simulink model "GPSModel"  (R2017a)
settings: Solver=VariableStepAuto  StartTime=0.0  StopTime=10.0  RelTol=1e-3
undefined symbols (not defined in the file or in its folder): dpsV1, dpsV1seed, dpsV2, dpsV2seed, dpsV3, dpsV3seed, dpsV4, dpsV4seed, dpsV5, dpsV5seed, dpsV6, dpsV6seed, GPS_CLK, GpsClockBias, GpsClockDrift, TDI0, VI0, XI0
libraries: simulink x6
settings Model: Creator=AHKh  LastModifiedBy=AHKh

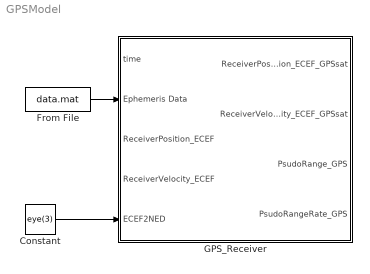
== system GPSModel ==
  Constant : Constant  Value=eye(3)
  From File : FromFile  FileName=data.mat  SampleTime=0
  GPS_Receiver : Subsystem
  wires:
  Constant/1 -> GPS_Receiver/5(ECEF2NED)
  From File/1 -> GPS_Receiver/2(Ephemeris Data)

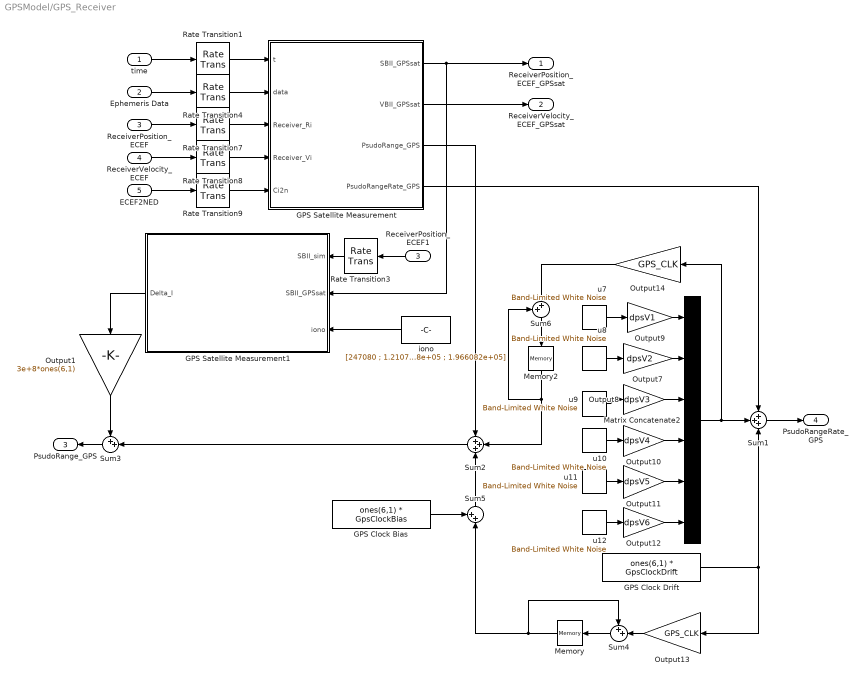
== system GPSModel/GPS_Receiver ==
  time : Inport  PortDimensions=[1,1]
  Ephemeris Data : Inport  Port=2
  ReceiverPosition_ECEF : Inport  Port=3  PortDimensions=[3,1]
  ReceiverVelocity_ECEF : Inport  Port=4  PortDimensions=[3,1]
  ECEF2NED : Inport  Port=5
  GPS Clock Bias : Constant  Value=ones(6,1) * GpsClockBias  VectorParams1D=off  SampleTime=GPS_CLK
  GPS Clock Drift : Constant  Value=ones(6,1) * GpsClockDrift  VectorParams1D=off  SampleTime=GPS_CLK
  GPS Satellite Measurement : MATLAB Function  TreatAsAtomicUnit=on
  GPS Satellite Measurement1 : MATLAB Function  TreatAsAtomicUnit=on
  Matrix Concatenate2 : Concatenate  NumInputs=6
  Memory : Memory  InheritSampleTime=on
  Memory2 : Memory  InheritSampleTime=on
  Output1 : Gain  Gain=3e+8*ones(6,1)  SaturateOnIntegerOverflow=on  OutDataTypeStr=Inherit: Same as input  ParamDataTypeStr=Inherit: Same as input
  Output10 : Gain  Gain=dpsV4  SaturateOnIntegerOverflow=on  OutDataTypeStr=Inherit: Same as input  ParamDataTypeStr=Inherit: Same as input
  Output11 : Gain  Gain=dpsV5  SaturateOnIntegerOverflow=on  OutDataTypeStr=Inherit: Same as input  ParamDataTypeStr=Inherit: Same as input
  Output12 : Gain  Gain=dpsV6  SaturateOnIntegerOverflow=on  OutDataTypeStr=Inherit: Same as input  ParamDataTypeStr=Inherit: Same as input
  Output13 : Gain  Gain=GPS_CLK  SaturateOnIntegerOverflow=on  OutDataTypeStr=Inherit: Same as input  ParamDataTypeStr=Inherit: Same as input
  Output14 : Gain  Gain=GPS_CLK  SaturateOnIntegerOverflow=on  OutDataTypeStr=Inherit: Same as input  ParamDataTypeStr=Inherit: Same as input
  Output7 : Gain  Gain=dpsV2  SaturateOnIntegerOverflow=on  OutDataTypeStr=Inherit: Same as input  ParamDataTypeStr=Inherit: Same as input
  Output8 : Gain  Gain=dpsV3  SaturateOnIntegerOverflow=on  OutDataTypeStr=Inherit: Same as input  ParamDataTypeStr=Inherit: Same as input
  Output9 : Gain  Gain=dpsV1  SaturateOnIntegerOverflow=on  OutDataTypeStr=Inherit: Same as input  ParamDataTypeStr=Inherit: Same as input
  Rate Transition1 : RateTransition  OutPortSampleTime=GPS_CLK
  Rate Transition3 : RateTransition  X0=XI0  OutPortSampleTime=GPS_CLK
  Rate Transition4 : RateTransition  OutPortSampleTime=GPS_CLK
  Rate Transition7 : RateTransition  X0=XI0  OutPortSampleTime=GPS_CLK
  Rate Transition8 : RateTransition  X0=VI0  OutPortSampleTime=GPS_CLK
  Rate Transition9 : RateTransition  X0=TDI0  OutPortSampleTime=GPS_CLK
  ReceiverPosition_ECEF1 : InportShadow  Port=3  PortDimensions=[3,1]
  Sum1 : Sum  Inputs=+++
  Sum2 : Sum  Inputs=+++
  Sum{3..6} (4 alike) : Sum  Inputs=++|
  iono : Constant  Value=[247080 ; 1.210719347000122e-08 ; -7.450580596923828e-09;-1.192092895507812e-07 ; 5.960464477539062e-08;9.6256e+04 ; -3.2768e+04 ; -1.96608e+05 ; 1.966082e+05]  VectorParams1D=off  SampleTime=GPS_CLK
  u10 : simulink/Sources/Band-Limited White Noise  Cov=[1]  Ts=GPS_CLK  seed=[dpsV4seed]
  u11 : simulink/Sources/Band-Limited White Noise  Cov=[1]  Ts=GPS_CLK  seed=[dpsV5seed]
  u12 : simulink/Sources/Band-Limited White Noise  Cov=[1]  Ts=GPS_CLK  seed=[dpsV6seed]
  u7 : simulink/Sources/Band-Limited White Noise  Cov=[1]  Ts=GPS_CLK  seed=[dpsV1seed]
  u8 : simulink/Sources/Band-Limited White Noise  Cov=[1]  Ts=GPS_CLK  seed=[dpsV2seed]
  u9 : simulink/Sources/Band-Limited White Noise  Cov=[1]  Ts=GPS_CLK  seed=[dpsV3seed]
  ReceiverPosition_ECEF_GPSsat : Outport
  ReceiverVelocity_ECEF_GPSsat : Outport  Port=2
  PsudoRange_GPS : Outport  Port=3
  PsudoRangeRate_GPS : Outport  Port=4
  wires:
  Rate Transition1/1 -> GPS Satellite Measurement/1(t)
  Rate Transition4/1 -> GPS Satellite Measurement/2(data)
  Rate Transition7/1 -> GPS Satellite Measurement/3(Receiver_Ri)
  Rate Transition8/1 -> GPS Satellite Measurement/4(Receiver_Vi)
  Rate Transition9/1 -> GPS Satellite Measurement/5(Ci2n)
  time/1 -> Rate Transition1/1
  GPS Satellite Measurement/1(SBII_GPSsat) -> ReceiverPosition_ECEF_GPSsat/1, GPS Satellite Measurement1/2(SBII_GPSsat)
  Ephemeris Data/1 -> Rate Transition4/1
  GPS Satellite Measurement/2(VBII_GPSsat) -> ReceiverVelocity_ECEF_GPSsat/1
  ReceiverPosition_ECEF/1 -> Rate Transition7/1
  ReceiverVelocity_ECEF/1 -> Rate Transition8/1
  ECEF2NED/1 -> Rate Transition9/1
  GPS Satellite Measurement/3(PsudoRange_GPS) -> Sum2/1
  u7/1 -> Output9/1
  Output9/1 -> Matrix Concatenate2/1
  u8/1 -> Output7/1
  Output7/1 -> Matrix Concatenate2/2
  u9/1 -> Output8/1
  Output8/1 -> Matrix Concatenate2/3
  u10/1 -> Output10/1
  Output10/1 -> Matrix Concatenate2/4
  u11/1 -> Output11/1
  Output11/1 -> Matrix Concatenate2/5
  u12/1 -> Output12/1
  Output12/1 -> Matrix Concatenate2/6
  Matrix Concatenate2/1 -> Output14/1, Sum1/2
  GPS Satellite Measurement/4(PsudoRangeRate_GPS) -> Sum1/1
  GPS Clock Drift/1 -> Sum1/3, Output13/1
  Memory/1 -> Sum4/1, Sum5/2
  Sum4/1 -> Memory/1
  Output13/1 -> Sum4/2
  Output14/1 -> Sum6/2
  Sum6/1 -> Memory2/1
  Memory2/1 -> Sum6/1, Sum2/2
  Sum5/1 -> Sum2/3
  GPS Clock Bias/1 -> Sum5/1
  Sum1/1 -> PsudoRangeRate_GPS/1
  ReceiverPosition_ECEF1/1 -> Rate Transition3/1
  iono/1 -> GPS Satellite Measurement1/3(iono)
  Sum2/1 -> Sum3/2
  GPS Satellite Measurement1/1(Delta_I) -> Output1/1
  Sum3/1 -> PsudoRange_GPS/1
  Rate Transition3/1 -> GPS Satellite Measurement1/1(SBII_sim)
  Output1/1 -> Sum3/1

== matlab function GPSModel/GPS_Receiver/GPS Satellite Measurement1 ==
  data: SBII_sim input; Delta_I output double; SBII_GPSsat input double; iono input
function Delta_I =Error_Ionospheric(SBII_sim,SBII_GPSsat,iono)
Pos_SV = SBII_GPSsat';
Pos_Rcv = SBII_sim';

GPS_Time=iono(1);
Alpha=iono(2:5);
Beta=iono(6:9);
% WGS84 ellipsoid constants:
a = 6378137;
e = 8.1819190842622e-2;
% calculations:
b   = sqrt(a^2*(1-e^2));
ep  = sqrt((a^2-b^2) / b^2);
p   = sqrt(Pos_Rcv(1)^2 + Pos_Rcv(2)^2);
th  = atan2(a*Pos_Rcv(3), b*p);
lon = atan2(Pos_Rcv(2) , Pos_Rcv(1));
lat = atan((Pos_Rcv(3) + ep^2*b*(sin(th))^3) / (p-e^2*a*(cos(th))^3));
N   = a/sqrt(1-e^2*(sin(lat))^2);
alt = p/cos(lat)-N;
% correct for numerical instability in altitude near exact poles:
% (after this correction, error is about 2 millimeters, which is about
% the same as the numerical precision of the overall function)
% k = abs(x)<1 & abs(y)<1;
% alt(k) = abs(z(k))-b;
GPS_Rcv = [lat,lon,alt];

Lat = GPS_Rcv(1)/pi;
Lon=GPS_Rcv(2)/pi;   % semicircles unit Lattitdue and Longitude 

E = zeros(6,1);
A = zeros(6,1);
F = zeros(6,1);
t = zeros(6,1);
x = zeros(6,1); 
Per = zeros(6,1);
AMP = zeros(6,1);
Psi = zeros(6,1);
Phi_L = zeros(6,1);
Phi_m = zeros(6,1);
Lambda_L = zeros(6,1);
T_iono = zeros(6,1);
for i=1:6 
    R = Pos_SV(i,:) - Pos_Rcv;               %vector from Reciever to Satellite
    Lat1 = GPS_Rcv(1);
    Lon1 = GPS_Rcv(2);
    XYZ2ENU=[-sin(Lon1) cos(Lon1) 0;...
           -sin(Lat1)*cos(Lon1) -sin(Lat1)*sin(Lon1) cos(Lat1);...
           cos(Lat1)*cos(Lon1) cos(Lat1)*sin(Lon1)  sin(Lat1)];...
    ENU=XYZ2ENU*R';  
  
    El = asin(ENU(3)/norm(ENU));
    A0 = atan2(ENU(1)/norm(ENU),ENU(2)/norm(ENU));

    E(i)=El/pi;                                            %SemiCircle Elevation
    A(i)=A0;                                               %SemiCircle Azimoth 
    % Calculate the Earth-Centered angle, Psi
    Psi(i)=0.0137/(E(i)+.11)-0.022;                        %SemiCircle

    %Compute the Subionospheric lattitude, Phi_L
    Phi_L(i)=Lat+Psi(i)*cos(A(i));                         %SemiCircle
    if Phi_L(i)>0.416
        Phi_L(i)=0.416;
    elseif Phi_L(i)<-0.416
        Phi_L(i)=-0.416;
    end

    %Compute the subionospheric longitude, Lambda_L
    Lambda_L(i)=Lon+(Psi(i)*sin(A(i))/cos(Phi_L(i)*pi));  %SemiCircle

    %Find the geomagnetic lattitude ,Phi_m, of the subionospheric location
    %looking toward each GPS satellite:
    Phi_m(i)=Phi_L(i)+0.064*cos((Lambda_L(i)-1.617)*pi);

    %Find the Local Time ,t, at the subionospheric point
    t(i)=4.23*10^4*Lambda_L(i)+GPS_Time;                 %GPS_Time(Sec)
    if t(i)>86400
        t(i)=t(i)-86400;
    elseif t(i)<0
        t(i)=t(i)+86400;
    end

    %Convert Slant time delay, Compute the Slant Factor,F
    F(i)=1+16*(.53-E(i)^3);

    %Compute the ionospheric time delay T_iono by first computing x
    Per(i)=Beta(1)+Beta(2)*Phi_m(i)+Beta(3)*Phi_m(i)^2+Beta(4)*Phi_m(i)^3;
    if Per(i) <72000                                     %Period
        Per(i)=72000;
    end
    x(i)=2*pi*(t(i)-50400)/Per(i);                       %Rad
    AMP(i)=Alpha(1)+Alpha(2)*Phi_m(i)+Alpha(3)*Phi_m(i)^2+Alpha(4)*Phi_m(i)^3;
    if AMP(i)<0 
        AMP(i) = 0;
    end
    if abs(x(i))>1.57
        T_iono(i)=F(i)*5*10^(-9);
    else
        T_iono(i)=F(i)*(5*10^(-9)+AMP(i)*(1-x(i)^2/2+x(i)^4/4));
    end

end%for

Delta_I=T_iono;

== matlab function GPSModel/GPS_Receiver/GPS Satellite Measurement ==
  data: t input; SBII_GPSsat output double; data input double; VBII_GPSsat output; Receiver_Ri input; Receiver_Vi input; Ci2n input; PsudoRange_GPS output; PsudoRangeRate_GPS output
function [SBII_GPSsat,VBII_GPSsat,PsudoRange_GPS,PsudoRangeRate_GPS] = position(t,data,Receiver_Ri,Receiver_Vi,Ci2n)
% This block supports the Embedded MATLAB subset.
% See the help menu for details. 
 eml.extrinsic('netraph')
% [Parameter,ST_NO]=size(data);

ST_NO = 28;
ST_NO1 = 28;

ST_NOf= 6;
Ri_GPS = zeros(3,ST_NO);
Vi_GPS = zeros(3,ST_NO);
SBII_GPSsat = zeros(3,ST_NOf);
VBII_GPSsat = zeros(3,ST_NOf);
PsudoRange_GPS = zeros(ST_NOf,1);
PsudoRangeRate_GPS = zeros(ST_NOf,1);

temp=0;
Elev= -2*ones(1,ST_NO1);
num=zeros(1,ST_NO1);
Azimuth=zeros(1,ST_NO1);
    
% Constant Parameter of this function
Mu=3.986005*10^14;
% Omega_dote = 7.2921151467*10^(-5);
ii=0;
% iii=0;jj=0;ST_Noi=0;

for ST_No=1:ST_NO

        A=data(7,ST_No)*data(7,ST_No);
        toe=data(8,ST_No);
        Delta_n=data(2,ST_No);
        M0=data(3,ST_No);
        omega=data(14,ST_No);
        C_us=data(6,ST_No);
        C_uc=data(4,ST_No);
        C_rs=data(1,ST_No);
        C_rc=data(13,ST_No);
        C_is=data(11,ST_No);
        C_ic=data(9,ST_No);
        i0=data(12,ST_No);
        IDOT=data(16,ST_No);
        Omega0=data(10,ST_No);
        Omegadot=data(15,ST_No);
        e=data(5,ST_No);

        %************************************************************************** 
        %************************************************************************** 
        %Compute Time From Ephemeris Refernce Epoch
        %Input:
            %t(sec):GPS Sys. Time
            %toe(sec):Reference Time Ephemeris
        %Output:
            %tk(sec):Time from ephemeris reference epoch
        tk=t-toe;
        %************************************************************************** 
        %************************************************************************** 
        %Compute corrected mean motion
        %Input:
            %A(meter): Semi-major axis
            %Mu(meter^3/sec^2): value of Earth's universal gravitational parameters
            %tk(sec):Time from Ephemeris Reference Epoch
            %Delta_n(semi-circle/sec):Mean Motion Diference From Computed Value
            %M0(semi-circles):
        %Output:
            %n0(Rad/sec):Computed mean motion 
            %n(semi-circle/sec):Corrected mean motion
            %Mk(semi-circle):Mean anomaly
        n0=sqrt(Mu/(A^3));
        n=n0/pi+Delta_n;
        Mk=M0+n*tk;

        %************************************************************************** 
        %************************************************************************** 
        %Solve Kepler Eq. with Initial value Ek0=Mk
        %Use Fzero Function to solve Kepler Eq.
        %The fzero command is an M-file. The algorithm, which was originated by 
        %T. Dekker, uses a combination of bisection, secant, and inverse quadratic
        %interpolation methods. An Algol 60 version, with some improvements, is 
        %given in [Brent, R., Algorithms for Minimization Without Derivatives, 
        %Prentice-Hall, 1973.]
        %Input:
            %Mk(semicircle): Mean Anomaly
            %e:  Eccentricity
        %Output:
            %Ek(Rad):  Eccentric Anomaly
%         Ek=1;
%         Ek=netraph(e,Mk*pi);
        % Ek=fzero(@(x) Kepler_Eq(x,Mk*pi,e),Mk*pi);
        Ek=0;
        arg=Mk*pi;
        %-----------------------
        B=cos(e)-(pi/2-e)*sin(e);
        E=arg+e*sin(arg)/(B+arg*sin(e));
        fE=E-e*sin(E)-arg;
        fpE=1-e*cos(E);
        dE=-fE/fpE;
        E=E+dE;
        while abs(fE)>1e-10
            fE=E-e*sin(E)-arg;
            fpE=1-e*cos(E);
            dE=-fE/fpE;
            E=E+dE;
        end
        Ek=E;
        %**************************************************************************
        %************************************************************************** 
        %Compute True Anomaly as a Function of Eccentric Anomaly
        %Input:
            %Ek(Rad):  Eccentric Anomaly
            %e      :  Eccentricity
        %Output:
            %nuk(Rad): True Anomaly
        Sin_nuk=sqrt(1-e^2)*sin(Ek)/(1-e*cos(Ek));
        Cos_nuk=(cos(Ek)-e)/(1-e*cos(Ek));
        nuk=atan2(Sin_nuk,Cos_nuk);
        if nuk<0
            nuk=nuk+2*pi;
        end
        %**************************************************************************
        %************************************************************************** 
        %Compute Argumet of Lattitude and Correction
        %Input:
            %nuk(Rad): True Anomaly
            %omega(semicircle):  Argument of perigee
        %Output:
            %Phik(Rad):  Argument of lattitude
        Phik=nuk+omega*pi;

        %**************************************************************************
        %************************************************************************** 
        %Compute Argumet of Lattitude,Radious and Inclination Correction
        %SEcond Harmonic Perturbation
        %Input:
            %Phik(Rad):  Argument of lattitude
            %C_us:Amplitude of the cosine harmonic correction term to the argument
            %     of lattitude(Rad)
            %C_uc:Amplitude of the sine harmonic correction term to the argument
            %     of lattitude(Rad)
            %C_rs:Amplitude of the cosine harmonic correction term to orbit
            %radius(meter)
            %C_rc:Amplitude of the sine harmonic correction term to orbit
            %radius(meter)
            %C_is:Amplitude of the cosine harmonic correction term to the angle of
            %     inclination(Rad)
            %C_ic:Amplitude of the sine harmonic correction term to the angle of
            %     inclination(Rad)
        %Output:
            % Delta_uk(Rad):Argument of lattitude correction
            % Delta_rk(meter):Argument of radius correction
            % Delta_ik(Rad):Argument of inclination correction

        Delta_uk=C_us*sin(2*Phik)+C_uc*cos(2*Phik);
        Delta_rk=C_rs*sin(2*Phik)+C_rc*cos(2*Phik);
        Delta_ik=C_is*sin(2*Phik)+C_ic*cos(2*Phik);
        %**************************************************************************
        %************************************************************************** 
        %Compute Corrected Value of Lattitude,Radious,Inclination and Ascendong
        %node
        %Input:
            % Phik(Rad):  Argument of lattitude
            % A(meter): Semi-major axis
            % Ek(Rad):  Eccentric Anomaly
            % e:  Eccentricity    
            % i0(semi-circle): inlination angle at reference time
            % Omega0(semi-circle): Refernce Longitude of Ascending Node
            % Omegadot(semi-circle/sec): rate of right ascension
            % Omega_dote(rad/sec):WGS 84 value of the earth's rotation rate
            % IDOT(semi-circle/sec): rate of inlination angle
            % Delta_uk(Rad):Argument of lattitude correction
            % Delta_rk(meter):Argument of radius correction
            % Delta_ik(Rad):Argument of inclination correction
        %Output:
            % uk(Rad):Corrcted argument of lattitude
            % rk(meter): corrected radius
            % ik(Rad):corrected inclination
            % Omegak(Rad):Corrected longitude of ascending node.
        uk=Phik+Delta_uk;              %Latitude
        rk=A*(1-e*cos(Ek))+Delta_rk;   %Radious
        ik=i0*pi+Delta_ik+IDOT*tk*pi;  %Inclination
        %  Omegak=Omega0*pi+(Omegadot*pi-Omega_dote)*tk-Omega_dote*toe;
         Omegak=Omega0*pi+(Omegadot*pi)*tk;
        %**************************************************************************
        %************************************************************************** 
        %Compute satellite vehicle position
        %Satellite position in orbital plane
        x_Perk=rk*cos(uk);
        y_Perk=rk*sin(uk);
        %Satellite velocity in orbital plane
        vx_Perk=-sqrt(Mu/(A*(1-e^2)))*sin(uk);
        vy_Perk=sqrt(Mu/(A*(1-e^2)))*(e+cos(uk));
        %Satellite Position in ECEF
        xk=x_Perk*cos(Omegak)-y_Perk*cos(ik)*sin(Omegak);
        yk=x_Perk*sin(Omegak)+y_Perk*cos(ik)*cos(Omegak);
        zk=y_Perk*sin(ik);
        %Satellite Velocity in ECEF
        vxk=vx_Perk*cos(Omegak)-vy_Perk*cos(ik)*sin(Omegak);
        vyk=vx_Perk*sin(Omegak)+vy_Perk*cos(ik)*cos(Omegak);
        vzk=vy_Perk*sin(ik);
        %Output:
            % xk,yk,zk(meter): Satellite Position in ECEF
            % Mk(semicircle): Mean Anomaly
            % Ek(Rad):  Eccentric Anomaly
            % nuk(Rad): True Anomaly
            % Phik(Rad):  Argument of lattitude
            % uk(Rad):Corrcted argument of lattitude
            % rk(meter): corrected radius
            % ik(Rad):corrected inclination
            % Omegak(Rad):Corrected longitude of ascending node.
            % A(meter):semi-major orbit axis
            % e: orbit eccentricity

        Ri_GPS(1,ST_No) = xk;
        Ri_GPS(2,ST_No) = yk;
        Ri_GPS(3,ST_No) = zk;
        %-------------
        Vi_GPS(1,ST_No) = vxk;
        Vi_GPS(2,ST_No) = vyk;
        Vi_GPS(3,ST_No) = vzk;
        
        PosDiffn = Ci2n * (Ri_GPS(:,ST_No)-Receiver_Ri);
                   
        Elevation = atan(-PosDiffn(3)/sqrt(PosDiffn(2)^2+PosDiffn(1)^2));
        
        if Elevation>10*pi/180,
           ii=ii+1; 
           num(ii)=ST_No;
           Elev(ii)=Elevation;
           Azimuth(ii)=atan2(PosDiffn(2),PosDiffn(1));
        end   
        
end

for iii=1:length(num)
    
    for jj=(iii+1):length(num)
          
        if Elev(iii)<Elev(jj), 
           temp=Elev(iii);
           Elev(iii)=Elev(jj);
           Elev(jj)=temp;
           temp=num(iii);
           num(iii)=num(jj);
           num(jj)=temp;
           temp= Azimuth(iii);
           Azimuth(iii)= Azimuth(jj);
           Azimuth(jj)=temp;
        end
    end
end


for ST_Noi=1:ST_NOf

        ST_No=num(ST_Noi);  
        SBII_GPSsat(1,ST_Noi) = Ri_GPS(1,ST_No);
        SBII_GPSsat(2,ST_Noi) = Ri_GPS(2,ST_No);
        SBII_GPSsat(3,ST_Noi) = Ri_GPS(3,ST_No);
    
        VBII_GPSsat(1,ST_Noi) = Vi_GPS(1,ST_No);
        VBII_GPSsat(2,ST_Noi) = Vi_GPS(2,ST_No);
        VBII_GPSsat(3,ST_Noi) = Vi_GPS(3,ST_No);
        
        PosDiff = SBII_GPSsat(:,ST_Noi) - Receiver_Ri;
        VelDiff = VBII_GPSsat(:,ST_Noi) - Receiver_Vi;

        PsudoRange_GPS(ST_Noi,1) = sqrt( PosDiff(1)^2 + PosDiff(2)^2 + PosDiff(3)^2 );
        PsudoRangeRate_GPS(ST_Noi,1) = dot(VelDiff,PosDiff) / PsudoRange_GPS(ST_Noi);
      
end
